simulink model "sim4"  (R2013a)
settings: Solver=ode45  StartTime=0.0  StopTime=10.0  RelTol=1e-3
values from neighbouring files (symbols this model uses):
  a0 = 6    [skrypt4.m]
  a1 = 3    [skrypt4.m]
  b = [4*qgn; 0]    [skrypt2.m]    (also in skrypt4.m = 2)
  czas_skoku = 0    [skrypt4.m]    (also in skrypt5.m = 2)
  du = 0')    [skrypt4.m]    (also in skrypt5.m = 0)
  u0 = 0    [skrypt4.m]    (also in skrypt5.m = 1)
  x0 = (-10/3)+b*u0/a0    (= -3.33333333333)    [skrypt4.m]    (also in skrypt5.m = tabx0(k))
settings Model: Creator=Junior  LastModifiedBy=Dawidek

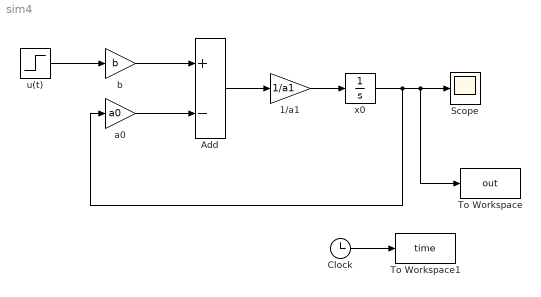
== system sim4 ==
  1/a1 : Gain  Gain=1/a1
  Add : Sum  Inputs=+-
  Clock : Clock
  Scope : Scope
  To Workspace : ToWorkspace  VariableName=out  SampleTime=-1
  To Workspace1 : ToWorkspace  VariableName=time  SampleTime=-1
  a0 : Gain  Gain=a0
  b : Gain  Gain=b
  u(t) : Step  Time=czas_skoku  Before=u0  After=u0+du  SampleTime=0
  x0 : Integrator  InitialCondition=x0
  wires:
  b/1 -> Add/1
  u(t)/1 -> b/1
  Add/1 -> 1/a1/1
  1/a1/1 -> x0/1
  x0/1 -> To Workspace/1, Scope/1, a0/1
  a0/1 -> Add/2
  Clock/1 -> To Workspace1/1
